simulink model "Reciver"  (R2020b)
settings: Solver=ode4  StartTime=0.0  StopTime=TF  FixedStep=h  RelTol=1e-3
values from neighbouring files (symbols this model uses):
  vR1 = -14600    [ReciverLocation.m]
  vR2 = vR1    (= -14600)    [ReciverLocation.m]
  x = 0    [ReciverLocation.m]
  xR1 = 1000000    [ReciverLocation.m]
  xR2 = 500000    [ReciverLocation.m]
  y = 0    [ReciverLocation.m]
  yR1 = KMtoFT(20000)    [ReciverLocation.m]
  yR2 = 500000    [ReciverLocation.m]
libraries: simulink x1, simulink_extras x1
settings Model: Creator=dariusmensah  LastModifiedBy=dariusmensah

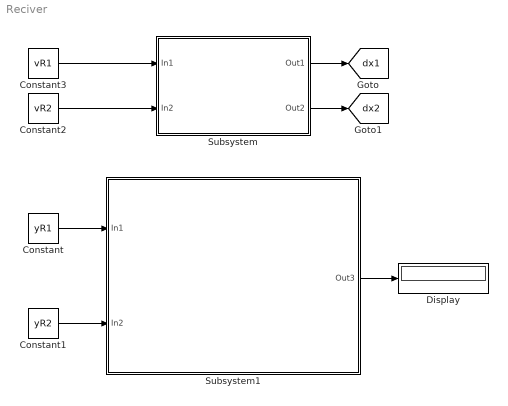
== system Reciver ==
  Constant : Constant  Value=yR1
  Constant1 : Constant  Value=yR2
  Constant2 : Constant  Value=vR2
  Constant3 : Constant  Value=vR1
  Display : Display
  Subsystem : Subsystem
  Subsystem1 : Subsystem
  tag scope: dx1=global, dx2=global
  wires:
  Constant3/1 -> Subsystem/1(In1)
  Constant2/1 -> Subsystem/2(In2)
  Subsystem/1(Out1) -> [dx1]
  Subsystem/2(Out2) -> [dx2]
  Constant/1 -> Subsystem1/1(In1)
  Constant1/1 -> Subsystem1/2(In2)
  Subsystem1/1(Out3) -> Display/1

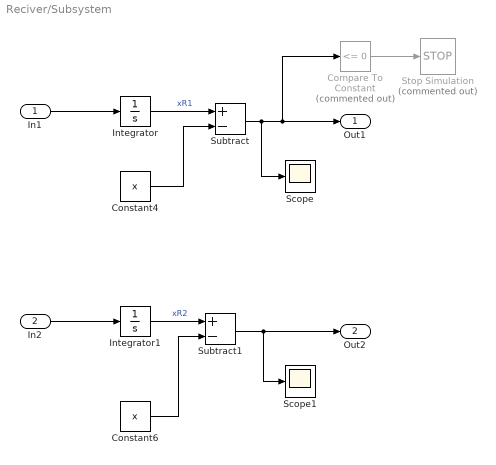
== system Reciver/Subsystem ==
  In1 : Inport
  In2 : Inport  Port=2
  Compare To Constant : simulink/Logic and Bit Operations/Compare To Constant  Commented=on  relop=<=  const=0  OutDataTypeStr=boolean
  Constant4 : Constant  Value=x
  Constant6 : Constant  Value=x
  Integrator : Integrator  InitialCondition=xR1
  Integrator1 : Integrator  InitialCondition=xR2
  Scope : Scope
  Scope1 : Scope
  Stop Simulation : Stop  Commented=on
  Subtract : Sum  Inputs=+-
  Subtract1 : Sum  Inputs=+-
  Out1 : Outport
  Out2 : Outport  Port=2
  wires:
  In2/1 -> Integrator1/1
  Subtract1/1 -> Scope1/1, Out2/1
  Subtract/1 -> Scope/1, Compare To Constant/1, Out1/1
  Integrator1/1 -> Subtract1/1  "xR2"
  In1/1 -> Integrator/1
  Constant4/1 -> Subtract/2
  Integrator/1 -> Subtract/1  "xR1"
  Constant6/1 -> Subtract1/2
  Compare To Constant/1 -> Stop Simulation/1

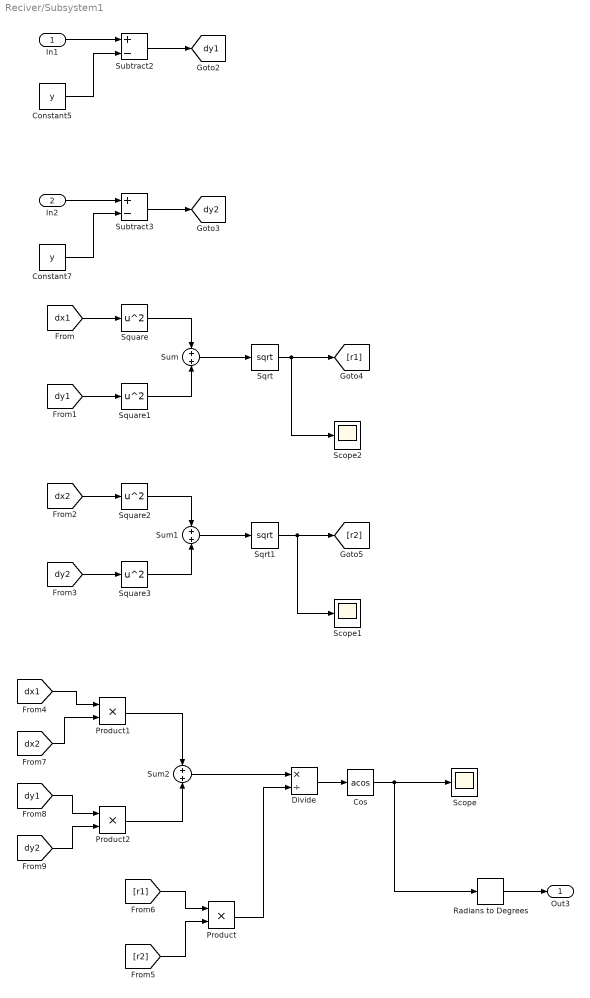
== system Reciver/Subsystem1 ==
  In1 : Inport
  In2 : Inport  Port=2
  Constant5 : Constant  Value=y
  Constant7 : Constant  Value=y
  Cos : Trigonometry  Operator=acos
  Divide : Product  Inputs=*/
  Product : Product
  Product1 : Product
  Product2 : Product
  Radians to Degrees : simulink_extras/Transformations/Radians to Degrees
  Scope : Scope
  Scope1 : Scope
  Scope2 : Scope
  Sqrt : Sqrt  SaturateOnIntegerOverflow=on
  Sqrt1 : Sqrt  SaturateOnIntegerOverflow=on
  Square{,1..3} (4 alike) : Math  Operator=square  SaturateOnIntegerOverflow=on
  Subtract2 : Sum  Inputs=+-
  Subtract3 : Sum  Inputs=+-
  Sum : Sum
  Sum1 : Sum
  Sum2 : Sum
  Out3 : Outport
  tag scope: dy1=global, dy2=global
  wires:
  [dy2] -> Square3/1
  Subtract2/1 -> [dy1]
  In2/1 -> Subtract3/1
  Constant7/1 -> Subtract3/2
  Sqrt/1 -> [r1], Scope2/1
  Sqrt1/1 -> [r2], Scope1/1
  Subtract3/1 -> [dy2]
  Constant5/1 -> Subtract2/2
  [dy1] -> Square1/1
  [dx1] -> Square/1
  Square/1 -> Sum/1
  [dx2] -> Square2/1
  Sum1/1 -> Sqrt1/1
  Square1/1 -> Sum/2
  Sum/1 -> Sqrt/1
  Square3/1 -> Sum1/2
  In1/1 -> Subtract2/1
  Square2/1 -> Sum1/1
  Sum2/1 -> Divide/1
  Product2/1 -> Sum2/2
  [dx1] -> Product1/1
  Product/1 -> Divide/2
  [dx2] -> Product1/2
  Product1/1 -> Sum2/1
  [dy1] -> Product2/1
  [dy2] -> Product2/2
  [r1] -> Product/1
  Radians to Degrees/1 -> Out3/1
  [r2] -> Product/2
  Divide/1 -> Cos/1
  Cos/1 -> Radians to Degrees/1, Scope/1
